simulink model "FDM_LPF_BPF"  (R2021a)
settings: Solver=VariableStepAuto  StartTime=0.0  StopTime=10.0  RelTol=1e-3
libraries: dsparch4 x10
settings Model: Creator=Bharat Gunhalkar  LastModifiedBy=Bharat Gunhalkar

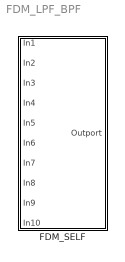
== system FDM_LPF_BPF ==
  FDM_SELF : Subsystem

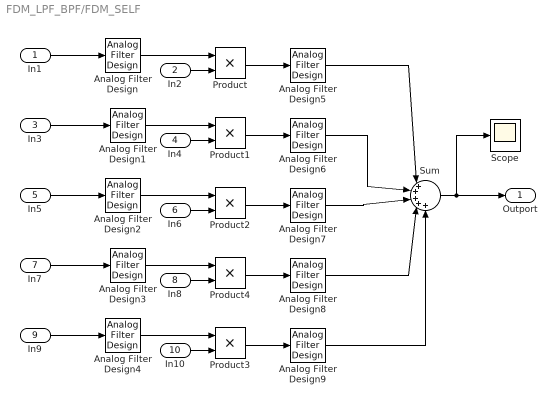
== system FDM_LPF_BPF/FDM_SELF ==
  In1 : Inport
  In2 : Inport  Port=2
  In3 : Inport  Port=3
  In4 : Inport  Port=4
  In5 : Inport  Port=5
  In6 : Inport  Port=6
  In7 : Inport  Port=7
  In8 : Inport  Port=8
  In9 : Inport  Port=9
  In10 : Inport  Port=10
  Analog Filter Design{,1..4} (5 alike) : dsparch4/Analog Filter Design  method=Butterworth  filttype=Lowpass  N=8  Wlo=30  Whi=80  Rp=2  Rs=40
  Analog Filter Design{5..9} (5 alike) : dsparch4/Analog Filter Design  method=Butterworth  filttype=Bandpass  N=8  Wlo=30  Whi=80  Rp=2  Rs=40
  Product{,1..4} (5 alike) : Product
  Scope : Scope
  Sum : Sum  Inputs=|+++++
  Outport : Outport
  wires:
  In3/1 -> Analog Filter Design1/1
  Analog Filter Design2/1 -> Product2/1
  Analog Filter Design6/1 -> Sum/2
  In5/1 -> Analog Filter Design2/1
  Analog Filter Design5/1 -> Sum/1
  In4/1 -> Product1/2
  Analog Filter Design3/1 -> Product4/1
  Analog Filter Design9/1 -> Sum/5
  Analog Filter Design1/1 -> Product1/1
  Product3/1 -> Analog Filter Design9/1
  In7/1 -> Analog Filter Design3/1
  Product/1 -> Analog Filter Design5/1
  Analog Filter Design/1 -> Product/1
  Product1/1 -> Analog Filter Design6/1
  Analog Filter Design8/1 -> Sum/4
  Analog Filter Design4/1 -> Product3/1
  In6/1 -> Product2/2
  Sum/1 -> Outport/1, Scope/1
  Product2/1 -> Analog Filter Design7/1
  Analog Filter Design7/1 -> Sum/3
  In2/1 -> Product/2
  In8/1 -> Product4/2
  In10/1 -> Product3/2
  Product4/1 -> Analog Filter Design8/1
  In1/1 -> Analog Filter Design/1
  In9/1 -> Analog Filter Design4/1
